simulink model "Preditor"  (R2019a)
settings: Solver=VariableStepAuto  StartTime=0.0  StopTime=10.0  RelTol=1e-3
values from neighbouring files (symbols this model uses):
  den = [1 50.1 275]    [pidpolyM.m]
  K = c1    [pidpolyM.m]
  num = 1500    [pidpolyM.m]
  Td = c2/K    [pidpolyM.m]
  Ti = K/c0    [pidpolyM.m]
libraries: simulink x3
settings Model: Creator=valte  LastModifiedBy=valte
settings SolverCC: AlgebraicLoopSolver=LineSearch

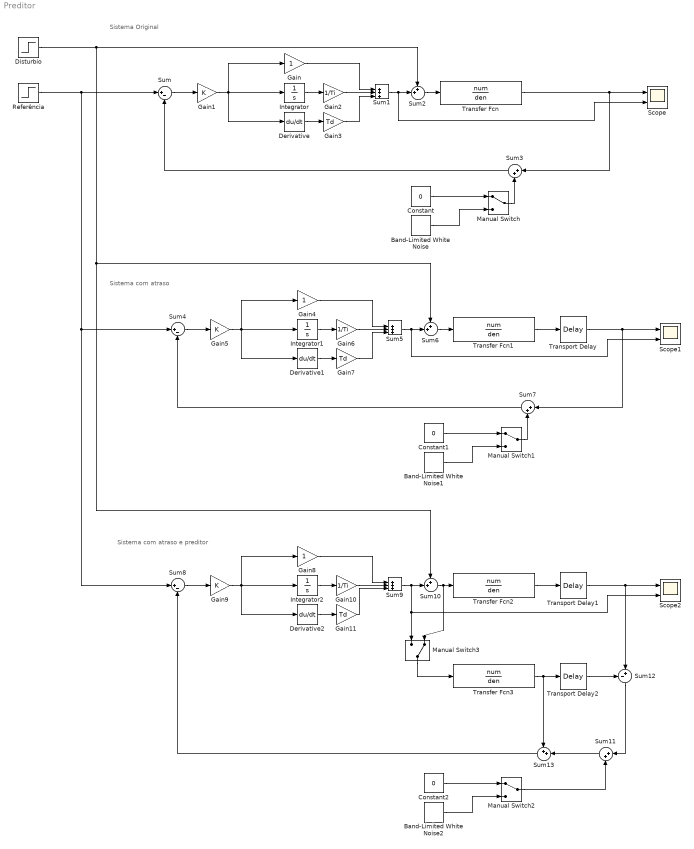
== system Preditor ==
  note: Sistema com atraso
  note: Sistema Original
  note: Sistema com atraso e preditor
  Band-Limited White Noise : simulink/Sources/Band-Limited White Noise  Cov=[0.1]  Ts=0.1  seed=[23341]
  Band-Limited White Noise1 : simulink/Sources/Band-Limited White Noise  Cov=[0.1]  Ts=0.1  seed=[23341]
  Band-Limited White Noise2 : simulink/Sources/Band-Limited White Noise  Cov=[0.1]  Ts=0.1  seed=[23341]
  Constant : Constant  Value=0
  Constant1 : Constant  Value=0
  Constant2 : Constant  Value=0
  Derivative : Derivative  CoefficientInTFapproximation=0.001
  Derivative1 : Derivative  CoefficientInTFapproximation=0.001
  Derivative2 : Derivative  CoefficientInTFapproximation=0.001
  Disturbio : Step  Time=4  After=.1  SampleTime=0
  Gain : Gain
  Gain1 : Gain  Gain=K
  Gain10 : Gain  Gain=1/Ti
  Gain11 : Gain  Gain=Td
  Gain2 : Gain  Gain=1/Ti
  Gain3 : Gain  Gain=Td
  Gain4 : Gain
  Gain5 : Gain  Gain=K
  Gain6 : Gain  Gain=1/Ti
  Gain7 : Gain  Gain=Td
  Gain8 : Gain
  Gain9 : Gain  Gain=K
  Integrator : Integrator
  Integrator1 : Integrator
  Integrator2 : Integrator
  Manual Switch : ManualSwitch
  Manual Switch1 : ManualSwitch
  Manual Switch2 : ManualSwitch
  Manual Switch3 : ManualSwitch  CurrentSetting=0
  Referência : Step  SampleTime=0
  Scope : Scope  NumInputPorts=2
  Scope1 : Scope  NumInputPorts=2
  Scope2 : Scope  NumInputPorts=2
  Sum : Sum  Inputs=|+-
  Sum1 : Sum  Inputs=|+++
  Sum{2,6,10,13} (4 alike) : Sum  Inputs=++|
  Sum11 : Sum  Inputs=|++
  Sum12 : Sum  Inputs=-+|
  Sum3 : Sum  Inputs=|++
  Sum4 : Sum  Inputs=|+-
  Sum5 : Sum  Inputs=|+++
  Sum7 : Sum  Inputs=|++
  Sum8 : Sum  Inputs=|+-
  Sum9 : Sum  Inputs=|+++
  Transfer Fcn{,1..3} (4 alike) : TransferFcn  Numerator=num  Denominator=den
  Transport Delay : TransportDelay  DelayTime=.2
  Transport Delay1 : TransportDelay  DelayTime=.5
  Transport Delay2 : TransportDelay  DelayTime=.5
  wires:
  Transfer Fcn/1 -> Sum3/1, Scope/1
  Sum/1 -> Gain1/1
  Gain1/1 -> Gain/1, Integrator/1, Derivative/1
  Gain/1 -> Sum1/1
  Gain2/1 -> Sum1/2
  Integrator/1 -> Gain2/1
  Derivative/1 -> Gain3/1
  Gain3/1 -> Sum1/3
  Sum2/1 -> Transfer Fcn/1
  Sum1/1 -> Scope/2, Sum2/2
  Sum3/1 -> Sum/2
  Manual Switch/1 -> Sum3/2
  Constant/1 -> Manual Switch/1
  Band-Limited White Noise/1 -> Manual Switch/2
  Sum5/1 -> Scope1/2, Sum6/2
  Derivative1/1 -> Gain7/1
  Gain6/1 -> Sum5/2
  Band-Limited White Noise1/1 -> Manual Switch1/2
  Gain5/1 -> Gain4/1, Integrator1/1, Derivative1/1
  Gain4/1 -> Sum5/1
  Constant1/1 -> Manual Switch1/1
  Sum4/1 -> Gain5/1
  Sum6/1 -> Transfer Fcn1/1
  Integrator1/1 -> Gain6/1
  Transfer Fcn1/1 -> Transport Delay/1
  Gain7/1 -> Sum5/3
  Sum7/1 -> Sum4/2
  Manual Switch1/1 -> Sum7/2
  Transport Delay/1 -> Sum7/1, Scope1/1
  Gain11/1 -> Sum9/3
  Manual Switch2/1 -> Sum11/2
  Transfer Fcn2/1 -> Transport Delay1/1
  Disturbio/1 -> Sum2/1, Sum6/1, Sum10/1
  Transport Delay1/1 -> Sum12/2, Scope2/1
  Integrator2/1 -> Gain10/1
  Constant2/1 -> Manual Switch2/1
  Sum8/1 -> Gain9/1
  Sum10/1 -> Manual Switch3/2, Transfer Fcn2/1
  Gain9/1 -> Gain8/1, Integrator2/1, Derivative2/1
  Referência/1 -> Sum8/1, Sum4/1, Sum/1
  Sum9/1 -> Scope2/2, Manual Switch3/1, Sum10/2
  Gain8/1 -> Sum9/1
  Gain10/1 -> Sum9/2
  Derivative2/1 -> Gain11/1
  Band-Limited White Noise2/1 -> Manual Switch2/2
  Transfer Fcn3/1 -> Sum13/1, Transport Delay2/1
  Manual Switch3/1 -> Transfer Fcn3/1
  Transport Delay2/1 -> Sum12/1
  Sum12/1 -> Sum11/1
  Sum11/1 -> Sum13/2
  Sum13/1 -> Sum8/2
